simulink model "SIM_SAD_DEMO"  (R2025b)
settings: Solver=ode5  StartTime=0.0  StopTime=T/10  FixedStep=0.1  RelTol=1e-3
model workspace (MAT data in the model file):
  Pnull : Simulink.Parameter (value not decoded)
  rho_albedo_medio : Simulink.Parameter (value not decoded)
values from neighbouring files (symbols this model uses):
  Aree = zeros(10,1)    [SCRIPT_SAD_DEMO.m]    (also in lab_7.m)
  c = astroConstants(5)*1e3    [SCRIPT_SAD_DEMO.m]    (also in lab_7.m)
  draan = 1.99096871e-7    (= 1.99096871e-07)    [SCRIPT_SAD_DEMO.m]
  eps_E = deg2rad(astroConstants(63))    [SCRIPT_SAD_DEMO.m]    (also in lab_7.m)
  F_e = 1358    [SCRIPT_SAD_DEMO.m]    (also in lab_7.m)
  j_B = [0.01; 0.05; 0.01]    [SCRIPT_SAD_DEMO.m]    (also in lab_7.m)
  J_depl = [100.9, 0, 0;           0, 25.1, 0;           0, 0, 91.6]*1e-2    [SCRIPT_SAD_DEMO.m]    (also in lab_7.m)
  JD0 = juliandate(startTime)    [SCRIPT_SAD_DEMO.m]
  kep = [a,e,incl,raan,w,theta]    [SCRIPT_SAD_DEMO.m]    (also in lab_7.m)
  mu = astroConstants(13)    [SCRIPT_SAD_DEMO.m]    (also in lab_7.m)
  n = sqrt( (mu/ (a)^3))    [SCRIPT_SAD_DEMO.m]    (also in lab_7.m = sqrt((mu/ ((a/1000)^3))))
  n_sun = 2*pi/T_sun    (= 1.99238499086e-07)    [SCRIPT_SAD_DEMO.m]    (also in lab_7.m)
  Nmat = [ ... (first row only)    [SCRIPT_SAD_DEMO.m]    (also in lab_7.m)
  r_sun = 1*AU    [SCRIPT_SAD_DEMO.m]    (also in lab_7.m = 1*ua)
  Re = astroConstants(23)    [SCRIPT_SAD_DEMO.m]    (also in lab_7.m)
  rf = [ ... (first row only)    [SCRIPT_SAD_DEMO.m]    (also in lab_7.m)
  rhod = 0.1*ones(10,1)    [SCRIPT_SAD_DEMO.m]    (also in lab_7.m)
  rhos = zeros(10,1)    [SCRIPT_SAD_DEMO.m]    (also in lab_7.m)
  theta = 0    [SCRIPT_SAD_DEMO.m]    (also in lab_7.m)
symbols that are objects in the model workspace (value not decoded): Pnull, rho_albedo_medio
undefined symbols (not defined in the file or in its folder): avec, bvec, DiscIntNeverNeededParam, dspblkCoreblockFVToolHelper, gcbh, Gyro, Magmeter, q, SRP, Sun_sensor
libraries: LIBRARY_SAD x37, matrix_library x28
(part 2 of 3)

== system SIM_SAD_DEMO/DCM->q (Shepperd Algorithm)/Normalized Vector1 ==
  r : Inport
  Constant : Constant  Value=1e-12
  Divide : Product  Inputs=*/
  Max : MinMax  Function=max  Inputs=2
  vector_norm : LIBRARY_SAD/vector_norm  SystemSampleTime=-1  VariantActivationTime=update diagram  EmptyChoice=off  PassThrough=off  PassThroughVariantControl=(default)  EmptyChoiceVariantControl=(default)  AllowFlexibleInterface=on  Latency=0  AutoFrameSizeCalculation=off
  r_norm : Outport
  wires:
  vector_norm/1 -> Max/1
  r/1 -> Divide/1, vector_norm/1
  Divide/1 -> r_norm/1
  Constant/1 -> Max/2
  Max/1 -> Divide/2

== system SIM_SAD_DEMO/DCM->q (Shepperd Algorithm)1/Normalized Vector1 ==
  r : Inport
  Constant : Constant  Value=1e-12
  Divide : Product  Inputs=*/
  Max : MinMax  Function=max  Inputs=2
  vector_norm : LIBRARY_SAD/vector_norm  SystemSampleTime=-1  VariantActivationTime=update diagram  EmptyChoice=off  PassThrough=off  PassThroughVariantControl=(default)  EmptyChoiceVariantControl=(default)  AllowFlexibleInterface=on  Latency=0  AutoFrameSizeCalculation=off
  r_norm : Outport
  wires:
  vector_norm/1 -> Max/1
  r/1 -> Divide/1, vector_norm/1
  Divide/1 -> r_norm/1
  Constant/1 -> Max/2
  Max/1 -> Divide/2

== system SIM_SAD_DEMO/DKE/ALBEDO_TORQUE ==
  note: Solar Radiation Pression Torque
  note: creo un blocco for each che mi permette di eseguire passo a passo ogni singola operazione del prodotto vettoriale, andando poi a crearmi il vettore uscita finale. In input ho un 10x3, però dentro il for each lavoro con delle 3x1 per semplicità, con vettori colonna quindi
  note: scarto i valori negativi perchè significa che mi trovo dalla parte opposta della faccia colpita dal sole, quindi non genero albedo, in quel caso tutto il satellite non viene colpito, quindi non mi serve creare una mask, ma basta semplicemente considerare il vettore nullo
  sun direction inertial : Inport
  Ab_n : Inport  Port=2
  S/C direction : Inport  Port=3
  Constant : Constant  Value=0
  Constant16 : Constant  Value=rf
  Constant2 : Constant  Value=Pnull
  Dot Product : DotProduct  OutDataTypeStr=Inherit: Inherit via internal rule
  For Each Subsystem1 : Subsystem  TreatAsAtomicUnit=on
  Matrix Multiply4 : Product  Multiplication=Matrix(*)
  Max : MinMax  Function=max  Inputs=2
  Normalization : Subsystem
  "Normalization " : Subsystem
  Normalization1 : Subsystem
  Reshape2 : Reshape  OutputDimensionality=Customize  OutputDimensions=[10 3]
  Ricavo i vettori forza1 : Subsystem
  Scope10 : Scope
      settings: ActiveDisplayYMinimum=-8805.2567998384475  ActiveDisplayYMaximum=8127.929464306656  DataLoggingVariableName=ScopeData17
  Scope9 : Scope
      settings: ActiveDisplayYMinimum=-9.2718061255302776E-25  ActiveDisplayYMaximum=2.6543612251060555E-24  DataLoggingVariableName=ScopeData25
  Sum of Elements2 : Sum  Inputs=+  CollapseMode=Specified dimension
  Switch : Switch  Criteria=u2 > Threshold  SaturateOnIntegerOverflow=off  InputSameDT=off
  To Workspace : ToWorkspace  VariableName=AlbRtorque  SampleTime=-1
  Transpose : Math  Operator=transpose
  Albedo_torque : Outport
  wires:
  Sum of Elements2/1 -> Transpose/1, To Workspace/1, Scope9/1
  Matrix Multiply4/1 -> Ricavo i vettori forza1/3(R_B), Normalization/1(In1)
  Normalization1/1(Out1) -> Dot Product/2
  Ricavo i vettori forza1/1(Out1) -> For Each Subsystem1/2(In2)
  For Each Subsystem1/1(Out1) -> Reshape2/1
  S/C direction/1 -> Scope10/1, Matrix Multiply4/2, Normalization1/1(R_N)
  "Normalization "/1(Out1) -> Dot Product/1
  Constant16/1 -> For Each Subsystem1/1(In1)
  Normalization/1(Out1) -> Ricavo i vettori forza1/1(" R_ B direction normalized")
  Dot Product/1 -> Max/1  "Illuminated"
  Ab_n/1 -> Matrix Multiply4/1
  sun direction inertial/1 -> "Normalization "/1(In1)
  Constant2/1 -> Switch/3
  Reshape2/1 -> Sum of Elements2/1
  Constant/1 -> Max/2
  Transpose/1 -> Switch/1
  Switch/1 -> Albedo_torque/1
  Max/1 -> Ricavo i vettori forza1/2(In2), [Illum]  "Illuminated"
  [Illum] -> Switch/2

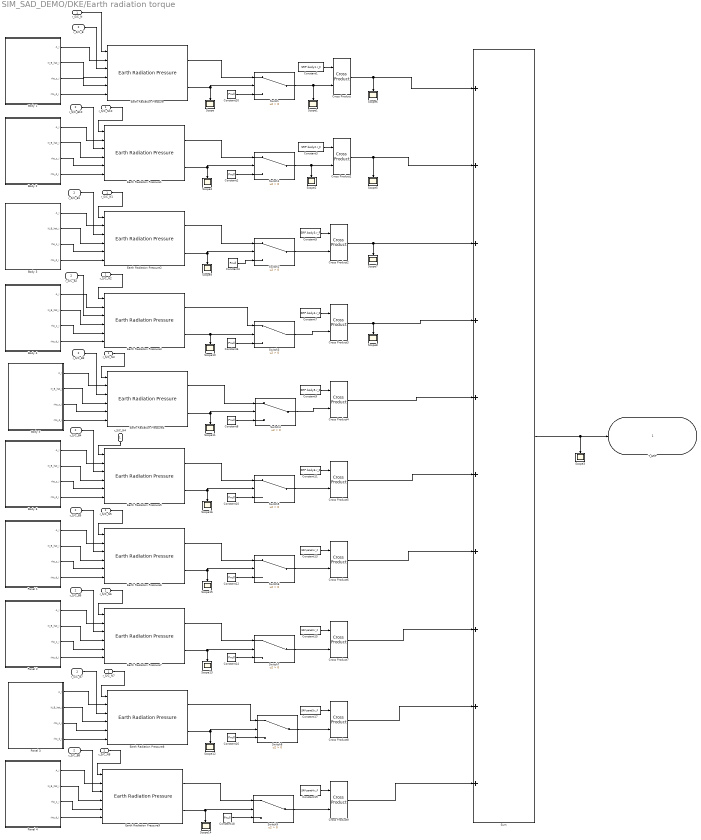
== system SIM_SAD_DEMO/DKE/Earth radiation torque ==
  r_S/C_N : Inport
  r_S/C_B : Inport  Port=2
  Body 1 : Subsystem
  Body 2 : Subsystem
  Body 3 : Subsystem
  Body 4 : Subsystem
  Body 5 : Subsystem
  Body 6 : Subsystem
  Constant1 : Constant  Value=SRP.body1.r_F
  Constant{2,4,6,8,10,12,14,16,18,20} (10 alike) : Constant  Value=Pnull
  Constant11 : Constant  Value=SRP.body6.r_F
  Constant13 : Constant  Value=SRP.panel1.r_F
  Constant15 : Constant  Value=SRP.panel2.r_F
  Constant17 : Constant  Value=SRP.panel3.r_F
  Constant19 : Constant  Value=SRP.panel4.r_F
  Constant3 : Constant  Value=SRP.body2.r_F
  Constant5 : Constant  Value=SRP.body3.r_F
  Constant7 : Constant  Value=SRP.body4.r_F
  Constant9 : Constant  Value=SRP.body5.r_F
  Cross Product{,1..9} (10 alike) : matrix_library/Cross Product
  Earth Radiation Pressure{,1..9} (10 alike) : LIBRARY_SAD/Earth Radiation Pressure  SystemSampleTime=-1  VariantActivationTime=update diagram  EmptyChoice=off  PassThrough=off  PassThroughVariantControl=(default)  EmptyChoiceVariantControl=(default)  AllowFlexibleInterface=on  Latency=0  AutoFrameSizeCalculation=off
  Panel 1 : Subsystem
  Panel 2 : Subsystem
  Panel 3 : Subsystem
  Panel 4 : Subsystem
  Scope{,1..16} (17 alike) : Scope
      Scope settings: ActiveDisplayYMinimum=-1  ActiveDisplayYMaximum=1  DataLoggingVariableName=ScopeData28
      Scope1 settings: ActiveDisplayYMinimum=-1  ActiveDisplayYMaximum=1  DataLoggingVariableName=ScopeData29
      Scope10 settings: DataLoggingVariableName=ScopeData11
      Scope11 settings: DataLoggingVariableName=ScopeData12
      Scope12 settings: DataLoggingVariableName=ScopeData13
      Scope13 settings: DataLoggingVariableName=ScopeData14
      Scope14 settings: DataLoggingVariableName=ScopeData15
      Scope15 settings: DataLoggingVariableName=ScopeData17
      Scope16 settings: DataLoggingVariableName=ScopeData18
      Scope2 settings: ActiveDisplayYMinimum=-1  ActiveDisplayYMaximum=1  DataLoggingVariableName=ScopeData30
      Scope3 settings: ActiveDisplayYMinimum=-5.1359030627651383E-25  ActiveDisplayYMaximum=9.2718061255302776E-25  DataLoggingVariableName=ScopeData31
      Scope4 settings: ActiveDisplayYMinimum=-1  ActiveDisplayYMaximum=1  DataLoggingVariableName=ScopeData32
      Scope5 settings: ActiveDisplayYMinimum=-1  ActiveDisplayYMaximum=1  DataLoggingVariableName=ScopeData33
      Scope6 settings: ActiveDisplayYMinimum=-1  ActiveDisplayYMaximum=1  DataLoggingVariableName=ScopeData34
      Scope7 settings: ActiveDisplayYMinimum=-1  ActiveDisplayYMaximum=1  DataLoggingVariableName=ScopeData35
      Scope8 settings: ActiveDisplayYMinimum=-1  ActiveDisplayYMaximum=1  DataLoggingVariableName=ScopeData36
      Scope9 settings: DataLoggingVariableName=ScopeData10
  Sum : Sum  Inputs=++++++++++
  Switch{,1..9} (10 alike) : Switch  Criteria=u2 > Threshold  SaturateOnIntegerOverflow=off  InputSameDT=off
  r_S/C_B{1..8,10} (9 alike) : InportShadow  Port=2
  r_S/C_N{1..8,10} (9 alike) : InportShadow
  T_ERP : Outport
  wires:
  Constant15/1 -> Cross Product7/1
  Switch6/1 -> Cross Product6/2
  Body 1/3(rho_s_i) -> Earth Radiation Pressure/5
  Constant6/1 -> Switch3/3
  Switch9/1 -> Cross Product9/2
  Constant13/1 -> Cross Product6/1
  Constant19/1 -> Cross Product9/1
  Cross Product4/1 -> Sum/5
  Constant16/1 -> Switch8/3
  Sum/1 -> Scope3/1, T_ERP/1
  Constant17/1 -> Cross Product8/1
  Constant1/1 -> Cross Product/1
  Switch5/1 -> Cross Product5/2
  r_S/C_B/1 -> Earth Radiation Pressure/3
  Switch3/1 -> Cross Product3/2
  Switch/1 -> Scope1/1, Cross Product/2
  Earth Radiation Pressure/2 -> Switch/2, Scope/1
  Cross Product9/1 -> Sum/10
  Cross Product3/1 -> Scope8/1, Sum/4
  Switch1/1 -> Scope2/1, Cross Product1/2
  Switch8/1 -> Cross Product8/2
  Cross Product2/1 -> Scope7/1, Sum/3
  Constant20/1 -> Switch/3
  Constant11/1 -> Cross Product5/1
  Constant8/1 -> Switch4/3
  Constant9/1 -> Cross Product4/1
  Earth Radiation Pressure/1 -> Switch/1
  Constant10/1 -> Switch5/3
  Switch4/1 -> Cross Product4/2
  Body 1/4(rho_d_i) -> Earth Radiation Pressure/6
  Cross Product5/1 -> Sum/6
  Constant3/1 -> Cross Product1/1
  Constant18/1 -> Switch9/3
  Constant14/1 -> Switch7/3
  Cross Product1/1 -> Sum/2, Scope5/1
  Constant2/1 -> Switch1/3
  Constant5/1 -> Cross Product2/1
  Constant12/1 -> Switch6/3
  Body 1/2(N_B_hat_i) -> Earth Radiation Pressure/4
  Cross Product6/1 -> Sum/7
  Body 1/1(A_i) -> Earth Radiation Pressure/2
  Cross Product7/1 -> Sum/8
  Switch2/1 -> Cross Product2/2
  Constant4/1 -> Switch2/3
  Switch7/1 -> Cross Product7/2
  Cross Product8/1 -> Sum/9
  Constant7/1 -> Cross Product3/1
  Cross Product/1 -> Scope6/1, Sum/1
  r_S/C_N/1 -> Earth Radiation Pressure/1
  Body 2/3(rho_s_i) -> Earth Radiation Pressure1/5
  Body 2/4(rho_d_i) -> Earth Radiation Pressure1/6
  Body 2/2(N_B_hat_i) -> Earth Radiation Pressure1/4
  r_S/C_B10/1 -> Earth Radiation Pressure1/3
  r_S/C_N10/1 -> Earth Radiation Pressure1/1
  Earth Radiation Pressure1/1 -> Switch1/1
  Earth Radiation Pressure1/2 -> Scope4/1, Switch1/2
  Body 2/1(A_i) -> Earth Radiation Pressure1/2
  Earth Radiation Pressure2/1 -> Switch2/1
  Body 3/2(N_B_hat_i) -> Earth Radiation Pressure2/4
  Body 3/4(rho_d_i) -> Earth Radiation Pressure2/6
  Body 3/1(A_i) -> Earth Radiation Pressure2/2
  Earth Radiation Pressure2/2 -> Scope9/1, Switch2/2
  r_S/C_N1/1 -> Earth Radiation Pressure2/1
  r_S/C_B1/1 -> Earth Radiation Pressure2/3
  Body 3/3(rho_s_i) -> Earth Radiation Pressure2/5
  Earth Radiation Pressure3/1 -> Switch3/1
  Body 4/2(N_B_hat_i) -> Earth Radiation Pressure3/4
  Body 4/4(rho_d_i) -> Earth Radiation Pressure3/6
  Body 4/1(A_i) -> Earth Radiation Pressure3/2
  Earth Radiation Pressure3/2 -> Switch3/2, Scope10/1
  r_S/C_N2/1 -> Earth Radiation Pressure3/1
  r_S/C_B2/1 -> Earth Radiation Pressure3/3
  Body 4/3(rho_s_i) -> Earth Radiation Pressure3/5
  Earth Radiation Pressure4/1 -> Switch4/1
  Body 5/2(N_B_hat_i) -> Earth Radiation Pressure4/4
  Body 5/4(rho_d_i) -> Earth Radiation Pressure4/6
  Body 5/1(A_i) -> Earth Radiation Pressure4/2
  Earth Radiation Pressure4/2 -> Scope11/1, Switch4/2
  r_S/C_N3/1 -> Earth Radiation Pressure4/1
  r_S/C_B3/1 -> Earth Radiation Pressure4/3
  Body 5/3(rho_s_i) -> Earth Radiation Pressure4/5
  Earth Radiation Pressure5/1 -> Switch5/1
  Body 6/2(N_B_hat_i) -> Earth Radiation Pressure5/4
  Body 6/4(rho_d_i) -> Earth Radiation Pressure5/6
  Body 6/1(A_i) -> Earth Radiation Pressure5/2
  Earth Radiation Pressure5/2 -> Scope16/1, Switch5/2
  r_S/C_N4/1 -> Earth Radiation Pressure5/1
  r_S/C_B4/1 -> Earth Radiation Pressure5/3
  Body 6/3(rho_s_i) -> Earth Radiation Pressure5/5
  Earth Radiation Pressure6/1 -> Switch6/1
  Panel 1/2(N_B_hat_i) -> Earth Radiation Pressure6/4
  Panel 1/4(rho_d_i) -> Earth Radiation Pressure6/6
  Panel 1/1(A_i) -> Earth Radiation Pressure6/2
  Earth Radiation Pressure6/2 -> Scope15/1, Switch6/2
  r_S/C_N5/1 -> Earth Radiation Pressure6/1
  r_S/C_B5/1 -> Earth Radiation Pressure6/3
  Panel 1/3(rho_s_i) -> Earth Radiation Pressure6/5
  Earth Radiation Pressure7/1 -> Switch7/1
  Panel 2/2(N_B_hat_i) -> Earth Radiation Pressure7/4
  Panel 2/4(rho_d_i) -> Earth Radiation Pressure7/6
  Panel 2/1(A_i) -> Earth Radiation Pressure7/2
  Earth Radiation Pressure7/2 -> Scope13/1, Switch7/2
  r_S/C_N6/1 -> Earth Radiation Pressure7/1
  r_S/C_B6/1 -> Earth Radiation Pressure7/3
  Panel 2/3(rho_s_i) -> Earth Radiation Pressure7/5
  Earth Radiation Pressure8/1 -> Switch8/1
  Panel 3/2(N_B_hat_i) -> Earth Radiation Pressure8/4
  Panel 3/4(rho_d_i) -> Earth Radiation Pressure8/6
  Panel 3/1(A_i) -> Earth Radiation Pressure8/2
  Earth Radiation Pressure8/2 -> Scope12/1, Switch8/2
  r_S/C_N7/1 -> Earth Radiation Pressure8/1
  r_S/C_B7/1 -> Earth Radiation Pressure8/3
  Panel 3/3(rho_s_i) -> Earth Radiation Pressure8/5
  Earth Radiation Pressure9/1 -> Switch9/1
  Panel 4/2(N_B_hat_i) -> Earth Radiation Pressure9/4
  Panel 4/4(rho_d_i) -> Earth Radiation Pressure9/6
  Panel 4/1(A_i) -> Earth Radiation Pressure9/2
  Earth Radiation Pressure9/2 -> Scope14/1, Switch9/2
  r_S/C_N8/1 -> Earth Radiation Pressure9/1
  r_S/C_B8/1 -> Earth Radiation Pressure9/3
  Panel 4/3(rho_s_i) -> Earth Radiation Pressure9/5

== system SIM_SAD_DEMO/DKE/Earth-S//C Orbit ==
  Keplerian Elements : Inport
  n : Inport  Port=2
  Conic Equation : Subsystem
  Constant1 : Constant
  Constant2 : Constant  Value=2
  Constant3 : Constant  Value=2
  Constant4 : Constant
  Constant5 : Constant  Value=3/2
  Cos : Trigonometry  Operator=cos
  Demux : Demux  Outputs=6
      settings: DisplayOption=none
  Divide1 : Product  Inputs=**/
  Gain{1..4} (4 alike) : Gain  Gain=pi/180
  Integrator : Integrator  InitialConditionSource=external  InitialCondition=theta  WrapState=on  WrappedStateUpperValue=2*pi  WrappedStateLowerValue=0
  Power : Math  Operator=pow
  Power1 : Math  Operator=pow
  Power2 : Math  Operator=pow
  Product1 : Product
  Sum : Sum
  Sum1 : Sum  Inputs=+-
  Sun-synchronous Orbit : Integrator  InitialConditionSource=external  WrapState=on  WrappedStateUpperValue=2*pi  WrappedStateLowerValue=0
  dRAAN_dt : Constant  Value=draan
  r (Inertial Frame) : Subsystem
  r_S/C_N : Outport
  theta_rad(t) : Outport  Port=2
  incl_rad : Outport  Port=3
  theta_dot : Outport  Port=4
  wires:
  Keplerian Elements/1 -> Demux/1
  Demux/1 -> Conic Equation/1(a)  "a"
  Demux/2 -> Product1/1, Power1/1, Conic Equation/2(e)  "e"
  Demux/3 -> Gain3/1  "incl"
  Demux/4 -> Gain2/1  "raan"
  Demux/5 -> Gain1/1  "w"
  Demux/6 -> Gain4/1  "theta"
  Constant1/1 -> Sum/1
  Cos/1 -> Product1/2
  Product1/1 -> Sum/2
  Sum/1 -> Power/1
  Constant2/1 -> Power/2
  Power/1 -> Divide1/2
  Constant3/1 -> Power1/2
  Power1/1 -> Sum1/2
  Constant4/1 -> Sum1/1
  Constant5/1 -> Power2/2
  Sum1/1 -> Power2/1
  Power2/1 -> Divide1/3
  Gain3/1 -> r (Inertial Frame)/3(incl_rad), incl_rad/1  "incl_rad"
  Gain2/1 -> Sun-synchronous Orbit/2  "raan_rad"
  Gain1/1 -> r (Inertial Frame)/5(w_rad)  "w_rad"
  r (Inertial Frame)/1(r_N) -> r_S/C_N/1
  n/1 -> Divide1/1
  Gain4/1 -> Integrator/2  "theta_rad"
  Conic Equation/1(r) -> r (Inertial Frame)/1(r)
  Integrator/1 -> Conic Equation/3(theta_rad(t)), theta_rad(t)/1, r (Inertial Frame)/2(theta_rad(t)), Cos/1  "theta_rad(t)"
  Divide1/1 -> Integrator/1, theta_dot/1  "theta_dot"
  dRAAN_dt/1 -> Sun-synchronous Orbit/1
  Sun-synchronous Orbit/1 -> r (Inertial Frame)/4(raan_rad)  "raan_rad"

== system SIM_SAD_DEMO/DKE/Gravity Gradient Torque ==
  I_matrix : Inport
  r_S/C_B : Inport  Port=2
  c_B : Inport  Port=3
  Constant : Constant  Value=3
  Constant1 : Constant  Value=mu
  Constant4 : Constant  Value=3
  Cross Product : matrix_library/Cross Product
  Divide : Product  Inputs=**/*
  MatrixMultiply : Product  Multiplication=Matrix(*)
  Power : Math  Operator=pow
  vector_norm : LIBRARY_SAD/vector_norm  SystemSampleTime=-1  VariantActivationTime=update diagram  EmptyChoice=off  PassThrough=off  PassThroughVariantControl=(default)  EmptyChoiceVariantControl=(default)  AllowFlexibleInterface=on  Latency=0  AutoFrameSizeCalculation=off
  T_GG : Outport
  wires:
  r_S/C_B/1 -> vector_norm/1
  Constant4/1 -> Power/2
  Constant/1 -> Divide/1
  Constant1/1 -> Divide/2
  Power/1 -> Divide/3
  I_matrix/1 -> MatrixMultiply/1
  c_B/1 -> MatrixMultiply/2, Cross Product/1
  MatrixMultiply/1 -> Cross Product/2
  Cross Product/1 -> Divide/4
  Divide/1 -> T_GG/1
  vector_norm/1 -> Power/1

== system SIM_SAD_DEMO/DKE/Kinematics (DCM) ==
  A_LVLH/N : Inport
  w_x : Inport  Port=2
  w_y : Inport  Port=3
  w_z : Inport  Port=4
  DCM Orthonormalisation : LIBRARY_SAD/DCM Orthonormalisation  SystemSampleTime=-1  VariantActivationTime=update diagram  EmptyChoice=off  PassThrough=off  PassThroughVariantControl=(default)  EmptyChoiceVariantControl=(default)  AllowFlexibleInterface=on  Latency=0  AutoFrameSizeCalculation=off
  DCM w matrix : LIBRARY_SAD/DCM w matrix  SystemSampleTime=-1  VariantActivationTime=update diagram  EmptyChoice=off  PassThrough=off  PassThroughVariantControl=(default)  EmptyChoiceVariantControl=(default)  AllowFlexibleInterface=on  Latency=0  AutoFrameSizeCalculation=off
  Gain : Gain  Gain=-1
  Integrator : Integrator  InitialConditionSource=external
  Product : Product  Multiplication=Matrix(*)
  To Workspace : ToWorkspace  VariableName=A_B_N  SampleTime=-1
  To Workspace1 : ToWorkspace  VariableName=A_B_N_ortho  SampleTime=-1
  A_B/N : Outport
  wires:
  A_LVLH/N/1 -> Integrator/2
  w_y/1 -> DCM w matrix/2
  w_z/1 -> DCM w matrix/3
  Integrator/1 -> To Workspace/1, DCM Orthonormalisation/1  "A_B/N"
  Product/1 -> Integrator/1  "A_dot"
  DCM w matrix/1 -> Gain/1
  w_x/1 -> DCM w matrix/1
  Gain/1 -> Product/1
  DCM Orthonormalisation/1 -> To Workspace1/1, A_B/N/1, Product/2  "A_B/N"

== system SIM_SAD_DEMO/DKE/Magnetic Torque ==
  A_B/N : Inport
  r_S/C_N : Inport  Port=2
  B_N (IGRF Model - Order N) : LIBRARY_SAD/B_N (IGRF Model - Order N)  SystemSampleTime=-1  VariantActivationTime=update diagram  EmptyChoice=off  PassThrough=off  PassThroughVariantControl=(default)  EmptyChoiceVariantControl=(default)  AllowFlexibleInterface=on  Latency=0  AutoFrameSizeCalculation=off
  Constant : Constant  Value=j_B
  Cross Product : matrix_library/Cross Product
  Display : Display
  IGRF magnetic torque : Subsystem
  MatrixMultiply : Product  Multiplication=Matrix(*)
  Scope : Scope
      settings: ActiveDisplayYMinimum=-1  ActiveDisplayYMaximum=1  DataLoggingVariableName=ScopeData5
  Scope1 : Scope
      settings: ActiveDisplayYMinimum=-1  ActiveDisplayYMaximum=1  DataLoggingVariableName=ScopeData22
  Scope13 : Scope
      settings: ActiveDisplayYMinimum=-1  ActiveDisplayYMaximum=1  DataLoggingVariableName=ScopeData37
  T_M : Outport
  B_N : Outport  Port=2
  wires:
  r_S/C_N/1 -> IGRF magnetic torque/1(r_S/C_N), B_N (IGRF Model - Order N)/1, Display/1
  A_B/N/1 -> MatrixMultiply/1
  MatrixMultiply/1 -> Scope/1, Cross Product/2  "B_B"
  Constant/1 -> Cross Product/1
  Cross Product/1 -> T_M/1
  B_N (IGRF Model - Order N)/1 -> B_N/1, MatrixMultiply/2, Scope1/1
  IGRF magnetic torque/1(B_ECI) -> Scope13/1

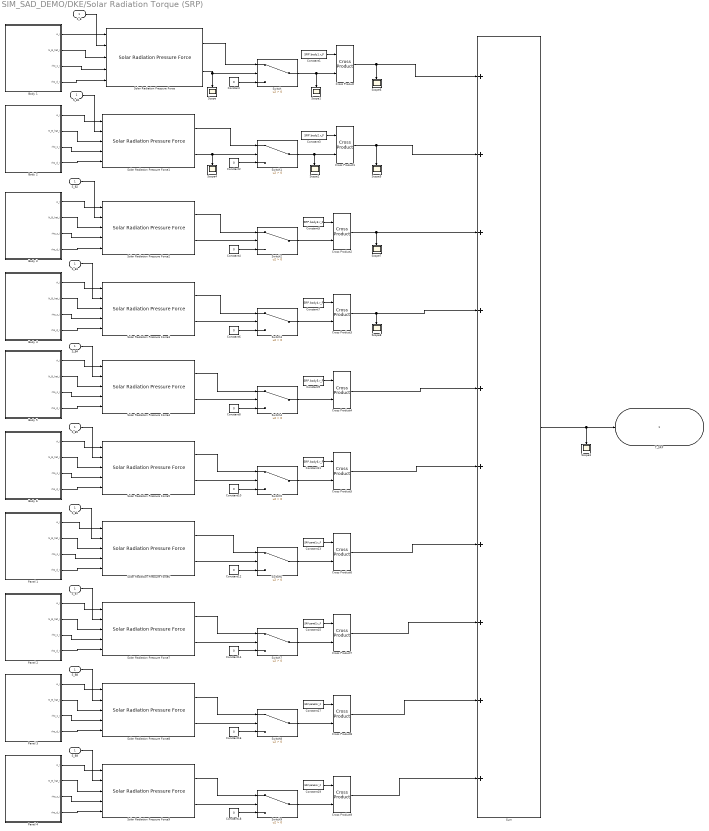
== system SIM_SAD_DEMO/DKE/Solar Radiation Torque (SRP) ==
  S_B : Inport
  Body 1 : Subsystem
  Body 2 : Subsystem
  Body 3 : Subsystem
  Body 4 : Subsystem
  Body 5 : Subsystem
  Body 6 : Subsystem
  Constant{,2,4,6,8,10,12,14,16,18} (10 alike) : Constant  Value=0
  Constant1 : Constant  Value=SRP.body1.r_F
  Constant11 : Constant  Value=SRP.body6.r_F
  Constant13 : Constant  Value=SRP.panel1.r_F
  Constant15 : Constant  Value=SRP.panel2.r_F
  Constant17 : Constant  Value=SRP.panel3.r_F
  Constant19 : Constant  Value=SRP.panel4.r_F
  Constant3 : Constant  Value=SRP.body2.r_F
  Constant5 : Constant  Value=SRP.body3.r_F
  Constant7 : Constant  Value=SRP.body4.r_F
  Constant9 : Constant  Value=SRP.body5.r_F
  Cross Product{,1..9} (10 alike) : matrix_library/Cross Product
  Panel 1 : Subsystem
  Panel 2 : Subsystem
  Panel 3 : Subsystem
  Panel 4 : Subsystem
  S_B{1..9} (9 alike) : InportShadow
  Scope{,1..8} (9 alike) : Scope
      Scope settings: ActiveDisplayYMinimum=-1  ActiveDisplayYMaximum=1  DataLoggingVariableName=ScopeData9
      Scope1 settings: ActiveDisplayYMinimum=-1  ActiveDisplayYMaximum=1  DataLoggingVariableName=ScopeData10
      Scope2 settings: ActiveDisplayYMinimum=-1  ActiveDisplayYMaximum=1  DataLoggingVariableName=ScopeData11
      Scope3 settings: ActiveDisplayYMinimum=-5.1359030627651383E-25  ActiveDisplayYMaximum=9.2718061255302776E-25  DataLoggingVariableName=ScopeData12
      Scope4 settings: ActiveDisplayYMinimum=-1  ActiveDisplayYMaximum=1  DataLoggingVariableName=ScopeData13
      Scope5 settings: ActiveDisplayYMinimum=-1  ActiveDisplayYMaximum=1  DataLoggingVariableName=ScopeData14
      Scope6 settings: ActiveDisplayYMinimum=-1  ActiveDisplayYMaximum=1  DataLoggingVariableName=ScopeData15
      Scope7 settings: ActiveDisplayYMinimum=-1  ActiveDisplayYMaximum=1  DataLoggingVariableName=ScopeData18
      Scope8 settings: ActiveDisplayYMinimum=-1  ActiveDisplayYMaximum=1  DataLoggingVariableName=ScopeData19
  Solar Radiation Pressure Force{,1..9} (10 alike) : LIBRARY_SAD/Solar Radiation Pressure Force  SystemSampleTime=-1  VariantActivationTime=update diagram  EmptyChoice=off  PassThrough=off  PassThroughVariantControl=(default)  EmptyChoiceVariantControl=(default)  AllowFlexibleInterface=on  Latency=0  AutoFrameSizeCalculation=off
  Sum : Sum  Inputs=++++++++++
  Switch{,1..9} (10 alike) : Switch  Criteria=u2 > Threshold  SaturateOnIntegerOverflow=off  InputSameDT=off
  T_SRP : Outport
  wires:
  S_B/1 -> Solar Radiation Pressure Force/2
  Body 1/1(A_i) -> Solar Radiation Pressure Force/1
  Body 1/2(N_B_hat_i) -> Solar Radiation Pressure Force/3
  Body 1/3(rho_s_i) -> Solar Radiation Pressure Force/4
  Body 1/4(rho_d_i) -> Solar Radiation Pressure Force/5
  Solar Radiation Pressure Force/1 -> Switch/1
  Solar Radiation Pressure Force/2 -> Scope/1, Switch/2
  Body 2/4(rho_d_i) -> Solar Radiation Pressure Force1/5
  Body 2/3(rho_s_i) -> Solar Radiation Pressure Force1/4
  Body 2/2(N_B_hat_i) -> Solar Radiation Pressure Force1/3
  Body 2/1(A_i) -> Solar Radiation Pressure Force1/1
  S_B1/1 -> Solar Radiation Pressure Force1/2
  S_B2/1 -> Solar Radiation Pressure Force2/2
  Body 3/1(A_i) -> Solar Radiation Pressure Force2/1
  Body 3/2(N_B_hat_i) -> Solar Radiation Pressure Force2/3
  Body 3/3(rho_s_i) -> Solar Radiation Pressure Force2/4
  Body 3/4(rho_d_i) -> Solar Radiation Pressure Force2/5
  Body 4/4(rho_d_i) -> Solar Radiation Pressure Force3/5
  Body 4/3(rho_s_i) -> Solar Radiation Pressure Force3/4
  Body 4/2(N_B_hat_i) -> Solar Radiation Pressure Force3/3
  Body 4/1(A_i) -> Solar Radiation Pressure Force3/1
  S_B3/1 -> Solar Radiation Pressure Force3/2
  S_B4/1 -> Solar Radiation Pressure Force4/2
  Body 5/1(A_i) -> Solar Radiation Pressure Force4/1
  Body 5/2(N_B_hat_i) -> Solar Radiation Pressure Force4/3
  Body 5/3(rho_s_i) -> Solar Radiation Pressure Force4/4
  Body 5/4(rho_d_i) -> Solar Radiation Pressure Force4/5
  Body 6/4(rho_d_i) -> Solar Radiation Pressure Force5/5
  Body 6/3(rho_s_i) -> Solar Radiation Pressure Force5/4
  Body 6/2(N_B_hat_i) -> Solar Radiation Pressure Force5/3
  Body 6/1(A_i) -> Solar Radiation Pressure Force5/1
  S_B5/1 -> Solar Radiation Pressure Force5/2
  S_B6/1 -> Solar Radiation Pressure Force6/2
  Panel 1/1(A_i) -> Solar Radiation Pressure Force6/1
  Panel 1/2(N_B_hat_i) -> Solar Radiation Pressure Force6/3
  Panel 1/3(rho_s_i) -> Solar Radiation Pressure Force6/4
  Panel 1/4(rho_d_i) -> Solar Radiation Pressure Force6/5
  Panel 2/4(rho_d_i) -> Solar Radiation Pressure Force7/5
  Panel 2/3(rho_s_i) -> Solar Radiation Pressure Force7/4
  Panel 2/2(N_B_hat_i) -> Solar Radiation Pressure Force7/3
  Panel 2/1(A_i) -> Solar Radiation Pressure Force7/1
  S_B7/1 -> Solar Radiation Pressure Force7/2
  S_B8/1 -> Solar Radiation Pressure Force8/2
  Panel 3/1(A_i) -> Solar Radiation Pressure Force8/1
  Panel 3/2(N_B_hat_i) -> Solar Radiation Pressure Force8/3
  Panel 3/3(rho_s_i) -> Solar Radiation Pressure Force8/4
  Panel 3/4(rho_d_i) -> Solar Radiation Pressure Force8/5
  Panel 4/4(rho_d_i) -> Solar Radiation Pressure Force9/5
  Panel 4/3(rho_s_i) -> Solar Radiation Pressure Force9/4
  Panel 4/2(N_B_hat_i) -> Solar Radiation Pressure Force9/3
  Panel 4/1(A_i) -> Solar Radiation Pressure Force9/1
  S_B9/1 -> Solar Radiation Pressure Force9/2
  Constant/1 -> Switch/3
  Switch/1 -> Scope1/1, Cross Product/2
  Constant1/1 -> Cross Product/1
  Cross Product/1 -> Scope6/1, Sum/1
  Cross Product1/1 -> Sum/2, Scope5/1
  Constant3/1 -> Cross Product1/1
  Switch1/1 -> Scope2/1, Cross Product1/2
  Constant2/1 -> Switch1/3
  Solar Radiation Pressure Force1/2 -> Scope4/1, Switch1/2
  Solar Radiation Pressure Force1/1 -> Switch1/1
  Solar Radiation Pressure Force2/1 -> Switch2/1
  Solar Radiation Pressure Force2/2 -> Switch2/2
  Constant4/1 -> Switch2/3
  Switch2/1 -> Cross Product2/2
  Constant5/1 -> Cross Product2/1
  Cross Product2/1 -> Scope7/1, Sum/3
  Cross Product3/1 -> Scope8/1, Sum/4
  Constant7/1 -> Cross Product3/1
  Switch3/1 -> Cross Product3/2
  Constant6/1 -> Switch3/3
  Solar Radiation Pressure Force3/2 -> Switch3/2
  Solar Radiation Pressure Force3/1 -> Switch3/1
  Solar Radiation Pressure Force4/1 -> Switch4/1
  Solar Radiation Pressure Force4/2 -> Switch4/2
  Constant8/1 -> Switch4/3
  Switch4/1 -> Cross Product4/2
  Constant9/1 -> Cross Product4/1
  Cross Product4/1 -> Sum/5
  Cross Product5/1 -> Sum/6
  Constant11/1 -> Cross Product5/1
  Switch5/1 -> Cross Product5/2
  Constant10/1 -> Switch5/3
  Solar Radiation Pressure Force5/2 -> Switch5/2
  Solar Radiation Pressure Force5/1 -> Switch5/1
  Solar Radiation Pressure Force6/1 -> Switch6/1
  Solar Radiation Pressure Force6/2 -> Switch6/2
  Constant12/1 -> Switch6/3
  Switch6/1 -> Cross Product6/2
  Constant13/1 -> Cross Product6/1
  Cross Product6/1 -> Sum/7
  Cross Product7/1 -> Sum/8
  Constant15/1 -> Cross Product7/1
  Switch7/1 -> Cross Product7/2
  Constant14/1 -> Switch7/3
  Solar Radiation Pressure Force7/2 -> Switch7/2
  Solar Radiation Pressure Force7/1 -> Switch7/1
  Solar Radiation Pressure Force8/1 -> Switch8/1
  Solar Radiation Pressure Force8/2 -> Switch8/2
  Constant16/1 -> Switch8/3
  Switch8/1 -> Cross Product8/2
  Constant17/1 -> Cross Product8/1
  Cross Product8/1 -> Sum/9
  Cross Product9/1 -> Sum/10
  Constant19/1 -> Cross Product9/1
  Switch9/1 -> Cross Product9/2
  Constant18/1 -> Switch9/3
  Solar Radiation Pressure Force9/2 -> Switch9/2
  Solar Radiation Pressure Force9/1 -> Switch9/1
  Sum/1 -> Scope3/1, T_SRP/1

== system SIM_SAD_DEMO/DKE/Sun-Earth Orbit ==
  Clock : Clock
  Clock1 : Clock
  Clock2 : Clock
  Constant : Constant  Value=n_sun
  Constant1 : Constant  Value=eps_E
  Constant2 : Constant  Value=r_sun
  Constant3 : Constant  Value=n_sun
  Constant4 : Constant  Value=eps_E
  Constant5 : Constant  Value=n_sun
  Cos : Trigonometry  Operator=cos
  Cos1 : Trigonometry  Operator=cos
  Cos2 : Trigonometry
  Product{,1..5} (6 alike) : Product
  Sin : Trigonometry
  Sin1 : Trigonometry
  Vector Concatenate : Concatenate  NumInputs=3
  r_Sun_N : Outport
  wires:
  Constant2/1 -> Product/1
  Clock/1 -> Product1/1
  Constant/1 -> Product1/2
  Product1/1 -> Cos/1
  Cos/1 -> Vector Concatenate/1
  Product2/1 -> Sin/1
  Constant3/1 -> Product2/2
  Clock1/1 -> Product2/1
  Sin/1 -> Product3/1
  Constant1/1 -> Cos1/1
  Product3/1 -> Vector Concatenate/2
  Cos1/1 -> Product3/2
  Cos2/1 -> Product5/2
  Product5/1 -> Vector Concatenate/3
  Constant4/1 -> Cos2/1
  Sin1/1 -> Product5/1
  Clock2/1 -> Product4/1
  Constant5/1 -> Product4/2
  Product4/1 -> Sin1/1
  Vector Concatenate/1 -> Product/2
  Product/1 -> r_Sun_N/1

== system SIM_SAD_DEMO/DKE/w_LVLH//N ==
  theta_dot : Inport
  Constant2 : Constant  Value=0
  Constant3 : Constant  Value=0
  Vector Concatenate1 : Concatenate  NumInputs=3
  Out1 : Outport
  wires:
  Vector Concatenate1/1 -> Out1/1  "w_LVLH/N"
  Constant2/1 -> Vector Concatenate1/1
  Constant3/1 -> Vector Concatenate1/2
  theta_dot/1 -> Vector Concatenate1/3

== system SIM_SAD_DEMO/SENSORS/Gyroscope ==
  note: misalignement e non-orthogonality
  note: Scale Factor Errors
  w_B (rad/s) : Inport
  Abs : Abs  SaturateOnIntegerOverflow=off
  Bias Instability (Brown noise) : RandomNumber  SampleTime=0.2
  Constant : Constant  Value=Gyro.R
  Constant1 : Constant  Value=Gyro.O
  Constant2 : Constant  Value=Gyro.b
  Constant3 : Constant  Value=0
  D2R : Gain  Gain=pi/180
  Discrete Transfer Fcn : DiscreteTransferFcn  Commented=on  LoadFcn=dspblkCoreblockFVToolHelper(gcbh,'load');
      settings: CopyFcn=dspblkCoreblockFVToolHelper(gcbh,'copy');  DeleteFcn=dspblkCoreblockFVToolHelper(gcbh,'close');  ModelCloseFcn=dspblkCoreblockFVToolHelper(gcbh,'close');  PreSaveFcn=dspblkCoreblockFVToolHelper(gcbh,'presave');  PostSaveFcn=dspblkCoreblockFVToolHelper(gcbh,'postsave');  CloseFcn=dspblkCoreblockFVToolHelper(gcbh,'close');
  Discrete-Time Integrator : DiscreteIntegrator  SampleTime=-1  ICPrevOutput=DiscIntNeverNeededParam  ICPrevScaledInput=DiscIntNeverNeededParam
  Gain2 : Gain  Gain=Gyro.D/(sqrt(2*Gyro.Ts))
  Gain3 : Gain  Commented=on  Gain=Gyro.D/(sqrt(2*Gyro.Ts))
  Gain4 : Gain  Gain=Gyro.D/(sqrt(2*Gyro.Ts))
  Gain5 : Gain  Gain=1/Gyro.ctime
  Gain6 : Gain  Gain=Gyro.SFN/100
  MatrixMultiply : Product  Multiplication=Matrix(*)
  MatrixMultiply2 : Product  Multiplication=Matrix(*)
  Minus : Sum  Inputs=+-
  Pink noise : RandomNumber  Commented=on  SampleTime=0.1
  Plus : Sum
  Plus1 : Sum  Inputs=+++
  Plus2 : Sum  Inputs=+++
  Quantizer : Quantizer  QuantizationInterval=Gyro.LSB
  R2D : Gain  Gain=180/pi
  R2D_1 : Gain  Gain=180/pi
  Saturation : Saturate  UpperLimit=Gyro.FS/2  LowerLimit=-Gyro.FS/2
  Scope{,1..6} (7 alike) : Scope
      Scope settings: ActiveDisplayYMinimum=-1  ActiveDisplayYMaximum=1  DataLoggingVariableName=ScopeData38
      Scope1 settings: ActiveDisplayYMinimum=-1  ActiveDisplayYMaximum=1  DataLoggingVariableName=ScopeData39
      Scope2 settings: ActiveDisplayYMinimum=-1  ActiveDisplayYMaximum=1  DataLoggingVariableName=ScopeData40
      Scope3 settings: ActiveDisplayYMinimum=-1  ActiveDisplayYMaximum=1  DataLoggingVariableName=ScopeData41
      Scope4 settings: ActiveDisplayYMinimum=-1  ActiveDisplayYMaximum=1  DataLoggingVariableName=ScopeData42
      Scope5 settings: ActiveDisplayYMinimum=-0.14265311547660356  ActiveDisplayYMaximum=1.1268108470363587  DataLoggingVariableName=ScopeData43
      Scope6 settings: ActiveDisplayYMinimum=-0.12498036504591503  ActiveDisplayYMaximum=1.124997818338435  DataLoggingVariableName=ScopeData44
  Square : Math  Operator=square
  Switch : Switch  Criteria=u2 > Threshold  Threshold=2*Gyro.NL*Gyro.FS  SaturateOnIntegerOverflow=off  InputSameDT=off
  White noise : RandomNumber  SampleTime=0.2
  Zero-Order Hold : ZeroOrderHold  SampleTime=Gyro.Ts
  w_m : Outport
  wires:
  w_B (rad/s)/1 -> MatrixMultiply/2, R2D_1/1
  MatrixMultiply/1 -> MatrixMultiply2/2
  Constant/1 -> MatrixMultiply/1, Scope5/1
  Constant1/1 -> Scope6/1, MatrixMultiply2/1
  MatrixMultiply2/1 -> R2D/1
  Constant2/1 -> Plus1/1
  Plus1/1 -> Scope4/1, Quantizer/1
  Quantizer/1 -> Saturation/1
  Saturation/1 -> D2R/1
  Zero-Order Hold/1 -> w_m/1
  D2R/1 -> Zero-Order Hold/1
  White noise/1 -> Gain2/1
  Bias Instability (Brown noise)/1 -> Gain4/1
  Gain3/1 -> Discrete Transfer Fcn/1
  Discrete Transfer Fcn/1 -> Plus2/3
  Gain2/1 -> Plus2/1, Scope2/1
  Gain4/1 -> Minus/1
  Minus/1 -> Discrete-Time Integrator/1
  Abs/1 -> Switch/2
  Square/1 -> Gain6/1
  Gain6/1 -> Switch/1
  Constant3/1 -> Switch/3
  R2D_1/1 -> Abs/1, Square/1
  Switch/1 -> Scope1/1, Plus/2
  Gain5/1 -> Minus/2
  Plus2/1 -> Scope3/1, Plus1/3
  Discrete-Time Integrator/1 -> Plus2/2, Gain5/1
  Plus/1 -> Plus1/2
  R2D/1 -> Plus/1, Scope/1
  Pink noise/1 -> Gain3/1

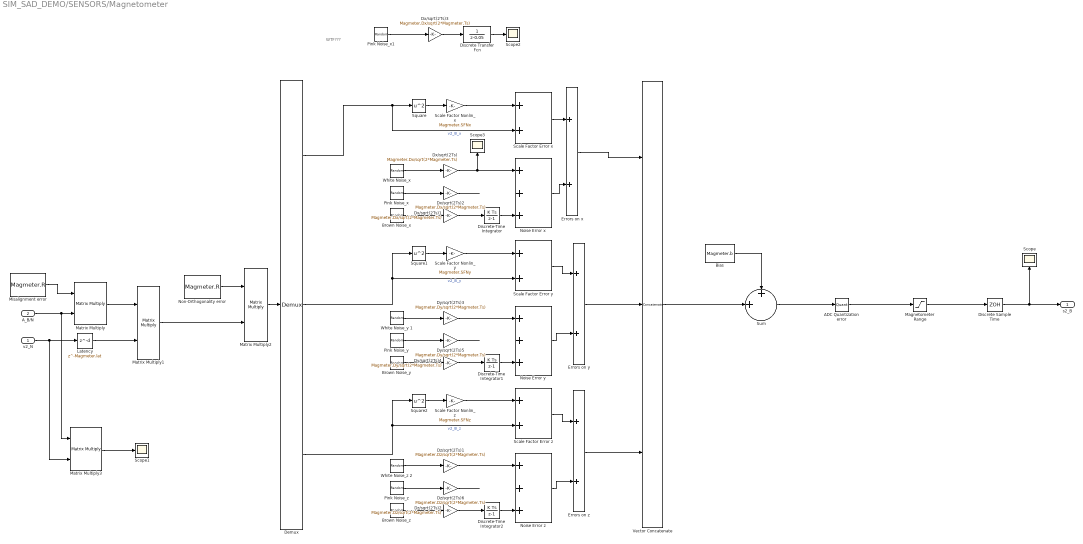
== system SIM_SAD_DEMO/SENSORS/Magnetometer ==
  note: WTF???
  v2_N : Inport
  A_B/N : Inport  Port=2
  ADC Quantization error : Quantizer  QuantizationInterval=Magmeter.LSB
  Bias : Constant  Value=Magmeter.b
  Brown Noise_x : RandomNumber  SampleTime=0.1
  Brown Noise_y : RandomNumber  SampleTime=0.1
  Brown Noise_z : RandomNumber  SampleTime=0.1
  Demux : Demux  Outputs=3
  Discrete Transfer Fcn : DiscreteTransferFcn  LoadFcn=dspblkCoreblockFVToolHelper(gcbh,'load');  Numerator=[1 ]  Denominator=[1 -0.05]
      settings: CopyFcn=dspblkCoreblockFVToolHelper(gcbh,'copy');  DeleteFcn=dspblkCoreblockFVToolHelper(gcbh,'close');  ModelCloseFcn=dspblkCoreblockFVToolHelper(gcbh,'close');  PreSaveFcn=dspblkCoreblockFVToolHelper(gcbh,'presave');  PostSaveFcn=dspblkCoreblockFVToolHelper(gcbh,'postsave');  CloseFcn=dspblkCoreblockFVToolHelper(gcbh,'close');
  Discrete Sample Time : ZeroOrderHold  SampleTime=Magmeter.Ts
  Discrete-Time Integrator : DiscreteIntegrator  SampleTime=-1  ICPrevOutput=DiscIntNeverNeededParam  ICPrevScaledInput=DiscIntNeverNeededParam
  Discrete-Time Integrator1 : DiscreteIntegrator  SampleTime=-1  ICPrevOutput=DiscIntNeverNeededParam  ICPrevScaledInput=DiscIntNeverNeededParam
  Discrete-Time Integrator2 : DiscreteIntegrator  SampleTime=-1  ICPrevOutput=DiscIntNeverNeededParam  ICPrevScaledInput=DiscIntNeverNeededParam
  Dx/sqrt(2Ts){,1..3} (4 alike) : Gain  Gain=Magmeter.Dx/sqrt(2*Magmeter.Ts)
  Dy/sqrt(2Ts)3 : Gain  Gain=Magmeter.Dy/sqrt(2*Magmeter.Ts)
  Dy/sqrt(2Ts)4 : Gain  Gain=Magmeter.Dy/sqrt(2*Magmeter.Ts)
  Dy/sqrt(2Ts)5 : Gain  Gain=Magmeter.Dy/sqrt(2*Magmeter.Ts)
  Dz/sqrt(2Ts)1 : Gain  Gain=Magmeter.Dz/sqrt(2*Magmeter.Ts)
  Dz/sqrt(2Ts)2 : Gain  Gain=Magmeter.Dz/sqrt(2*Magmeter.Ts)
  Dz/sqrt(2Ts)6 : Gain  Gain=Magmeter.Dz/sqrt(2*Magmeter.Ts)
  Errors on x : Sum
  Errors on y : Sum
  Errors on z : Sum
  Latency : Delay  DelayLength=Magmeter.lat
  Magnetometer Range : Saturate  UpperLimit=Magmeter.FS(2)  LowerLimit=Magmeter.FS(1)
  Matrix Multiply{,1..3} (4 alike) : Product  Multiplication=Matrix(*)
  Misalignment error : Constant  Value=Magmeter.R
  Noise Error x : Sum  Inputs=+++
  Noise Error y : Sum  Inputs=+++
  Noise Error z : Sum  Inputs=+++
  Non-Orthogonality error : Constant  Value=Magmeter.R
  Pink Noise_x : RandomNumber  SampleTime=0.1
  Pink Noise_x1 : RandomNumber  SampleTime=0.1
  Pink Noise_y : RandomNumber  SampleTime=0.1
  Pink Noise_z : RandomNumber  SampleTime=0.1
  Scale Factor Error x : Sum
  Scale Factor Error y : Sum
  Scale Factor Error z : Sum
  Scale Factor Nonlin_x : Gain  Gain=Magmeter.SFNx
  Scale Factor Nonlin_y : Gain  Gain=Magmeter.SFNy
  Scale Factor Nonlin_z : Gain  Gain=Magmeter.SFNz
  Scope{,1..3} (4 alike) : Scope
      Scope settings: ActiveDisplayYMinimum=-2.19268798828125E-5  ActiveDisplayYMaximum=3.19366455078125E-5  DataLoggingVariableName=ScopeData41
      Scope1 settings: ActiveDisplayYMinimum=-2.3197965857438213E-5  ActiveDisplayYMaximum=2.9408763146413098E-5  DataLoggingVariableName=ScopeData51
      Scope2 settings: ActiveDisplayYMinimum=-2.2418910951791633E-7  ActiveDisplayYMaximum=2.2323509891367277E-7  DataLoggingVariableName=ScopeData58
      Scope3 settings: ActiveDisplayYMinimum=-2.2049299467588538E-7  ActiveDisplayYMaximum=2.2303254095659386E-7  DataLoggingVariableName=ScopeData59
  Square : Math  Operator=square
  Square1 : Math  Operator=square
  Square2 : Math  Operator=square
  Sum : Sum  Inputs=++|
  Vector Concatenate : Concatenate  NumInputs=3
  "White Noise_x " : RandomNumber  SampleTime=0.1
  White Noise_y 1 : RandomNumber  SampleTime=0.1
  White Noise_z 2 : RandomNumber  SampleTime=0.1
  s2_B : Outport
  wires:
  v2_N/1 -> Matrix Multiply3/2, Latency/1
  A_B/N/1 -> Matrix Multiply3/1, Matrix Multiply/2
  Matrix Multiply/1 -> Matrix Multiply1/1
  Misalignment error/1 -> Matrix Multiply/1
  Latency/1 -> Matrix Multiply1/2
  Matrix Multiply1/1 -> Matrix Multiply2/2
  Non-Orthogonality error/1 -> Matrix Multiply2/1
  Matrix Multiply2/1 -> Demux/1
  Demux/1 -> Square/1, Scale Factor Error x/2  "v2_B_x"
  Demux/2 -> Square1/1, Scale Factor Error y/2  "v2_B_y"
  "White Noise_x "/1 -> Dx/sqrt(2Ts)/1
  Square/1 -> Scale Factor Nonlin_x/1
  Scale Factor Nonlin_x/1 -> Scale Factor Error x/1
  Noise Error x/1 -> Errors on x/2
  Scale Factor Error x/1 -> Errors on x/1
  Bias/1 -> Sum/1
  Errors on x/1 -> Vector Concatenate/1
  Vector Concatenate/1 -> Sum/2
  Sum/1 -> ADC Quantization error/1
  ADC Quantization error/1 -> Magnetometer Range/1
  Magnetometer Range/1 -> Discrete Sample Time/1
  Discrete Sample Time/1 -> s2_B/1, Scope/1
  Pink Noise_x/1 -> Dx/sqrt(2Ts)2/1
  Brown Noise_x/1 -> Dx/sqrt(2Ts)1/1
  Discrete-Time Integrator/1 -> Noise Error x/3
  Dx/sqrt(2Ts)1/1 -> Discrete-Time Integrator/1
  Demux/3 -> Scale Factor Error z/2, Square2/1  "v2_B_z"
  Dy/sqrt(2Ts)4/1 -> Discrete-Time Integrator1/1
  Discrete-Time Integrator1/1 -> Noise Error y/3
  Brown Noise_y/1 -> Dy/sqrt(2Ts)4/1
  Pink Noise_y/1 -> Dy/sqrt(2Ts)5/1
  Errors on y/1 -> Vector Concatenate/2
  Dy/sqrt(2Ts)3/1 -> Noise Error y/1
  Scale Factor Error y/1 -> Errors on y/1
  Noise Error y/1 -> Errors on y/2
  Scale Factor Nonlin_y/1 -> Scale Factor Error y/1
  Square1/1 -> Scale Factor Nonlin_y/1
  White Noise_y 1/1 -> Dy/sqrt(2Ts)3/1
  White Noise_z 2/1 -> Dz/sqrt(2Ts)1/1
  Square2/1 -> Scale Factor Nonlin_z/1
  Scale Factor Nonlin_z/1 -> Scale Factor Error z/1
  Noise Error z/1 -> Errors on z/2
  Scale Factor Error z/1 -> Errors on z/1
  Dz/sqrt(2Ts)1/1 -> Noise Error z/1
  Errors on z/1 -> Vector Concatenate/3
  Pink Noise_z/1 -> Dz/sqrt(2Ts)6/1
  Brown Noise_z/1 -> Dz/sqrt(2Ts)2/1
  Discrete-Time Integrator2/1 -> Noise Error z/3
  Dz/sqrt(2Ts)2/1 -> Discrete-Time Integrator2/1
  Matrix Multiply3/1 -> Scope1/1
  ? -> Noise Error z/2
  Dz/sqrt(2Ts)6/1 -> ?
  Dx/sqrt(2Ts)3/1 -> Discrete Transfer Fcn/1
  Discrete Transfer Fcn/1 -> Scope2/1
  ? -> Noise Error x/2
  Dx/sqrt(2Ts)2/1 -> ?
  Dx/sqrt(2Ts)/1 -> Scope3/1, Noise Error x/1
  Pink Noise_x1/1 -> Dx/sqrt(2Ts)3/1
  Dy/sqrt(2Ts)5/1 -> ?
  ? -> Noise Error y/2

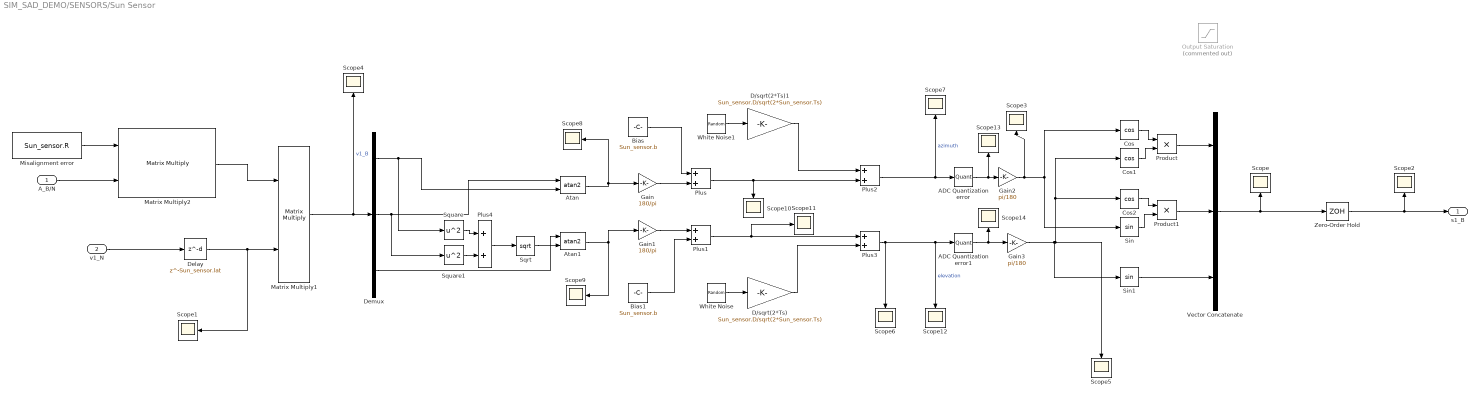
== system SIM_SAD_DEMO/SENSORS/Sun Sensor ==
  A_B/N : Inport
  v1_N : Inport  Port=2
  ADC Quantization error : Quantizer  QuantizationInterval=Sun_sensor.LSB
  ADC Quantization error1 : Quantizer  QuantizationInterval=Sun_sensor.LSB
  Atan : Trigonometry  Operator=atan2
  Atan1 : Trigonometry  Operator=atan2
  Bias : Constant  Value=Sun_sensor.b
  Bias1 : Constant  Value=Sun_sensor.b
  Cos : Trigonometry  Operator=cos
  Cos1 : Trigonometry  Operator=cos
  Cos2 : Trigonometry  Operator=cos
  D/sqrt(2*Ts) : Gain  Gain=Sun_sensor.D/sqrt(2*Sun_sensor.Ts)
  D/sqrt(2*Ts)1 : Gain  Gain=Sun_sensor.D/sqrt(2*Sun_sensor.Ts)
  Delay : Delay  DelayLength=Sun_sensor.lat
  Demux : Demux  Outputs=3
  Gain : Gain  Gain=180/pi
  Gain1 : Gain  Gain=180/pi
  Gain2 : Gain  Gain=pi/180
  Gain3 : Gain  Gain=pi/180
  Matrix Multiply1 : Product  Multiplication=Matrix(*)
  Matrix Multiply2 : Product  Multiplication=Matrix(*)
  Misalignment error : Constant  Value=Sun_sensor.R
  Output Saturation : Saturate  Commented=on  UpperLimit=Sun_sensor.FOV(2)  LowerLimit=Sun_sensor.FOV(1)
  Plus{,1..4} (5 alike) : Sum
  Product : Product
  Product1 : Product
  Scope{,1..14} (15 alike) : Scope
      Scope settings: ActiveDisplayYMinimum=-1.2499999209761798  ActiveDisplayYMaximum=1.2499998658254696  DataLoggingVariableName=ScopeData38
      Scope1 settings: ActiveDisplayYMinimum=-0.50368682988878122  ActiveDisplayYMaximum=0.83961433978529221  DataLoggingVariableName=ScopeData39
      Scope10 settings: ActiveDisplayYMinimum=-1  ActiveDisplayYMaximum=1  DataLoggingVariableName=ScopeData48
      Scope11 settings: ActiveDisplayYMinimum=-0.16263647893928282  ActiveDisplayYMaximum=0.22803548611194213  DataLoggingVariableName=ScopeData49
      Scope12 settings: ActiveDisplayYMinimum=-1  ActiveDisplayYMaximum=1  DataLoggingVariableName=ScopeData50
      Scope13 settings: ActiveDisplayYMinimum=-225.30372619628906  ActiveDisplayYMaximum=225.44471740722656  DataLoggingVariableName=ScopeData53
      Scope14 settings: ActiveDisplayYMinimum=-0.908203125  ActiveDisplayYMaximum=0.95947265625  DataLoggingVariableName=ScopeData54
      Scope2 settings: ActiveDisplayYMinimum=-1.0615675808468883  ActiveDisplayYMaximum=1.1316838676859093  DataLoggingVariableName=ScopeData40
      Scope3 settings: ActiveDisplayYMinimum=-3.91845703125  ActiveDisplayYMaximum=3.91845703125  DataLoggingVariableName=ScopeData43
      Scope4 settings: ActiveDisplayYMinimum=-1.2500019852403355  ActiveDisplayYMaximum=1.2500020169480639  DataLoggingVariableName=ScopeData42
      Scope5 settings: ActiveDisplayYMinimum=-0.015851134808151625  ActiveDisplayYMaximum=0.01674595693441825  DataLoggingVariableName=ScopeData52
      Scope6 settings: ActiveDisplayYMinimum=-1  ActiveDisplayYMaximum=1  DataLoggingVariableName=ScopeData44
      Scope7 settings: ActiveDisplayYMinimum=-225.01352290442006  ActiveDisplayYMaximum=225.27088940788934  DataLoggingVariableName=ScopeData45
      Scope8 settings: ActiveDisplayYMinimum=-3.6715953390719882  ActiveDisplayYMaximum=3.318983817677017  DataLoggingVariableName=ScopeData46
      Scope9 settings: ActiveDisplayYMinimum=-1  ActiveDisplayYMaximum=1  DataLoggingVariableName=ScopeData47
  Sin : Trigonometry
  Sin1 : Trigonometry
  Sqrt : Sqrt
  Square : Math  Operator=square
  Square1 : Math  Operator=square
  Vector Concatenate : Concatenate  NumInputs=3
  White Noise : RandomNumber  SampleTime=0.1
  White Noise1 : RandomNumber  SampleTime=0.1
  Zero-Order Hold : ZeroOrderHold  SampleTime=Sun_sensor.Ts
  s1_B : Outport
  wires:
  A_B/N/1 -> Matrix Multiply2/2
  Zero-Order Hold/1 -> s1_B/1, Scope2/1
  Vector Concatenate/1 -> Zero-Order Hold/1, Scope/1
  v1_N/1 -> Delay/1
  Misalignment error/1 -> Matrix Multiply2/1
  White Noise/1 -> D/sqrt(2*Ts)/1
  Bias/1 -> Plus/1
  Matrix Multiply1/1 -> Scope4/1, Demux/1  "v1_B"
  Atan/1 -> Scope8/1, Gain/1
  Atan1/1 -> Gain1/1, Scope9/1
  Delay/1 -> Matrix Multiply1/2, Scope1/1
  Gain/1 -> Plus/2
  Gain1/1 -> Plus1/1
  Plus/1 -> Plus2/2, Scope10/1
  Plus1/1 -> Scope11/1, Plus3/1
  D/sqrt(2*Ts)/1 -> Plus3/2
  Bias1/1 -> Plus1/2
  White Noise1/1 -> D/sqrt(2*Ts)1/1
  D/sqrt(2*Ts)1/1 -> Plus2/1
  Demux/3 -> Atan1/1
  Demux/1 -> Square/1, Atan/2
  Product/1 -> Vector Concatenate/1
  Demux/2 -> Square1/1, Atan/1
  Square1/1 -> Plus4/2
  Square/1 -> Plus4/1
  Plus4/1 -> Sqrt/1
  Sqrt/1 -> Atan1/2
  Cos/1 -> Product/1
  Cos1/1 -> Product/2
  ADC Quantization error/1 -> Gain2/1, Scope13/1
  ADC Quantization error1/1 -> Gain3/1, Scope14/1
  Sin1/1 -> Vector Concatenate/3
  Cos2/1 -> Product1/1
  Sin/1 -> Product1/2
  Product1/1 -> Vector Concatenate/2
  Plus3/1 -> Scope6/1, ADC Quantization error1/1, Scope12/1  "elevation"
  Plus2/1 -> ADC Quantization error/1, Scope7/1  "azimuth"
  Matrix Multiply2/1 -> Matrix Multiply1/1
  Gain2/1 -> Scope3/1, Cos/1, Sin/1
  Gain3/1 -> Scope5/1, Cos2/1, Cos1/1, Sin1/1

== system SIM_SAD_DEMO/q-->DCM/[qΛ] ==
  q : Inport
  Constant : Constant  Value=0
  Constant1 : Constant  Value=0
  Constant2 : Constant  Value=0
  Demux : Demux
  Gain : Gain  Gain=-1
  Gain1 : Gain  Gain=-1
  Gain2 : Gain  Gain=-1
  Terminator : Terminator
  Vector Concatenate : Concatenate  NumInputs=3
  Vector Concatenate1 : Concatenate  NumInputs=3  Mode=Multidimensional array  ConcatenateDimension=2
  Vector Concatenate2 : Concatenate  NumInputs=3
  Vector Concatenate3 : Concatenate  NumInputs=3
  "[qΛ]" : Outport
  wires:
  q/1 -> Demux/1
  Demux/1 -> Gain2/1, Vector Concatenate2/3  "q1"
  Demux/2 -> Vector Concatenate3/1, Gain/1  "q2"
  Demux/3 -> Vector Concatenate/2, Gain1/1  "q3"
  Demux/4 -> Terminator/1  "q4"
  Constant/1 -> Vector Concatenate/1
  Gain/1 -> Vector Concatenate/3
  Vector Concatenate/1 -> Vector Concatenate1/1
  Constant1/1 -> Vector Concatenate2/2
  Gain1/1 -> Vector Concatenate2/1
  Vector Concatenate2/1 -> Vector Concatenate1/2
  Gain2/1 -> Vector Concatenate3/2
  Constant2/1 -> Vector Concatenate3/3
  Vector Concatenate3/1 -> Vector Concatenate1/3
  Vector Concatenate1/1 -> "[qΛ]"/1

== system SIM_SAD_DEMO/ATTITUDE DETERMINATION (q-method)/w_est (q)/Normalized Vector ==
  r : Inport
  Divide : Product  Inputs=*/
  vector_norm : LIBRARY_SAD/vector_norm  SystemSampleTime=-1  VariantActivationTime=update diagram  EmptyChoice=off  PassThrough=off  PassThroughVariantControl=(default)  EmptyChoiceVariantControl=(default)  AllowFlexibleInterface=on  Latency=0  AutoFrameSizeCalculation=off
  s1_B : Outport
  wires:
  Divide/1 -> s1_B/1
  r/1 -> Divide/1, vector_norm/1
  vector_norm/1 -> Divide/2

== system SIM_SAD_DEMO/DCM ---> q/q-->DCM (CHECK)/[qΛ] ==
  q : Inport
  Constant : Constant  Value=0
  Constant1 : Constant  Value=0
  Constant2 : Constant  Value=0
  Demux : Demux
  Gain : Gain  Gain=-1
  Gain1 : Gain  Gain=-1
  Gain2 : Gain  Gain=-1
  Terminator : Terminator
  Vector Concatenate : Concatenate  NumInputs=3
  Vector Concatenate1 : Concatenate  NumInputs=3  Mode=Multidimensional array  ConcatenateDimension=2
  Vector Concatenate2 : Concatenate  NumInputs=3
  Vector Concatenate3 : Concatenate  NumInputs=3
  "[qΛ]" : Outport
  wires:
  Vector Concatenate1/1 -> "[qΛ]"/1
  Vector Concatenate3/1 -> Vector Concatenate1/3
  Constant2/1 -> Vector Concatenate3/3
  Gain2/1 -> Vector Concatenate3/2
  Vector Concatenate2/1 -> Vector Concatenate1/2
  Gain1/1 -> Vector Concatenate2/1
  Constant1/1 -> Vector Concatenate2/2
  Vector Concatenate/1 -> Vector Concatenate1/1
  Gain/1 -> Vector Concatenate/3
  Constant/1 -> Vector Concatenate/1
  Demux/4 -> Terminator/1  "q4"
  Demux/3 -> Gain1/1, Vector Concatenate/2  "q3"
  Demux/2 -> Gain/1, Vector Concatenate3/1  "q2"
  Demux/1 -> Vector Concatenate2/3, Gain2/1  "q1"
  q/1 -> Demux/1

== system SIM_SAD_DEMO/DKE/ALBEDO_TORQUE/For Each Subsystem1 ==
  note: nelle proprietà lascio direttamente così almeno posso processare una alla volta le singole righe e colonne sia in dimension che in width
  In1 : Inport  Partition=on  PartitionDimension=1  PartitionWidth=1  PartitionOffset=0
  In2 : Inport  Port=2  Partition=on  PartitionDimension=1  PartitionWidth=1  PartitionOffset=0
  Cross Product : matrix_library/Cross Product
  For Each : ForEach  DisableCoverage=on
  Signal Specification : SignalSpecification  Dimensions=[1 3]
  Transpose : Math  Operator=transpose
  Transpose1 : Math  Operator=transpose
  Transpose2 : Math  Operator=transpose
  Out1 : Outport  ConcatenationDimension=1
  wires:
  In2/1 -> Transpose/1  "Rfi"
  In1/1 -> Transpose1/1  "Fi"
  Transpose/1 -> Cross Product/1
  Transpose1/1 -> Cross Product/2
  Cross Product/1 -> Transpose2/1
  Transpose2/1 -> Signal Specification/1
  Signal Specification/1 -> Out1/1

== system SIM_SAD_DEMO/DKE/ALBEDO_TORQUE/Normalization ==
  In1 : Inport
  Divide : Product  Inputs=*/
  Dot Product : DotProduct  OutDataTypeStr=Inherit: Inherit via internal rule
  Sqrt : Sqrt
  Out1 : Outport
  wires:
  Dot Product/1 -> Sqrt/1
  In1/1 -> Divide/1, Dot Product/2, Dot Product/1
  Divide/1 -> Out1/1
  Sqrt/1 -> Divide/2

== system SIM_SAD_DEMO/DKE/ALBEDO_TORQUE/Normalization  ==
  In1 : Inport
  Divide : Product  Inputs=*/
  Dot Product : DotProduct  OutDataTypeStr=Inherit: Inherit via internal rule
  Sqrt : Sqrt
  Out1 : Outport
  wires:
  Dot Product/1 -> Sqrt/1
  In1/1 -> Divide/1, Dot Product/2, Dot Product/1
  Divide/1 -> Out1/1
  Sqrt/1 -> Divide/2

== system SIM_SAD_DEMO/DKE/ALBEDO_TORQUE/Normalization1 ==
  R_N : Inport
  Divide : Product  Inputs=*/
  Dot Product : DotProduct  OutDataTypeStr=Inherit: Inherit via internal rule
  Sqrt : Sqrt
  Out1 : Outport
  wires:
  Dot Product/1 -> Sqrt/1
  R_N/1 -> Divide/1, Dot Product/2, Dot Product/1
  Divide/1 -> Out1/1
  Sqrt/1 -> Divide/2
